simulink model "cameraCar_cs_mohammad"  (R2017b)
settings: Solver=ode5  StartTime=0.0  StopTime=inf  FixedStep=1/200  RelTol=1e-3
PreLoadFcn:
  | mbxruntime.callbacks.PreLoadFcn(bdroot);
PostLoadFcn:
  | mbxruntime.callbacks.PostLoadFcn(bdroot);
InitFcn:
  | mbxruntime.callbacks.InitFcn(bdroot);
StartFcn:
  | mbxruntime.callbacks.StartFcn(bdroot);
StopFcn:
  | mbxruntime.callbacks.StopFcn(bdroot);
model workspace (MAT data in the model file):
  mbox_table : struct (value not decoded)
  model_closed = 0
  sim_status = 0
undefined symbols (not defined in the file or in its folder): DiscIntNeverNeededParam, warningInitialVelocity, x0
libraries: simulink x19, dspnetwork x9, etargetslib x8, simulink_extras x5, PreScanSimulinkLibrary x4
(part 4 of 4)

== system cameraCar_cs_mohammad/Toyota_Yaris_Hatchback_1/Dynamics_Simple/Chassis/Bicycle_model_[XYZ]/Y & Yaw_Motion/Configurable Subsystem ==
  In1 : Inport
  In2 : Inport  Port=2
  Integrator : Integrator  ExternalReset=level
  Out1 : Outport
  wires:
  In1/1 -> Integrator/1
  In2/1 -> Integrator/2
  Integrator/1 -> Out1/1

== system cameraCar_cs_mohammad/Toyota_Yaris_Hatchback_1/Dynamics_Simple/Chassis/Bicycle_model_[XYZ]/Y & Yaw_Motion/Configurable Subsystem1 ==
  In1 : Inport
  Integrator : Integrator
  Out1 : Outport
  wires:
  In1/1 -> Integrator/1
  Integrator/1 -> Out1/1

== system cameraCar_cs_mohammad/Toyota_Yaris_Hatchback_1/Dynamics_Simple/Chassis/Bicycle_model_[XYZ]/Y & Yaw_Motion/Configurable Subsystem2 ==
  In1 : Inport
  In2 : Inport  Port=2
  Integrator : Integrator  ExternalReset=level
  Out1 : Outport
  wires:
  In1/1 -> Integrator/1
  In2/1 -> Integrator/2
  Integrator/1 -> Out1/1

== system cameraCar_cs_mohammad/Toyota_Yaris_Hatchback_1/Dynamics_Simple/Chassis/Bicycle_model_[XYZ]/Z, Pitch_Motion & Roll_Motion/Configurable Subsystem ==
  In1 : Inport
  Integrator : Integrator  LimitOutput=on  UpperSaturationLimit=5*pi/180  LowerSaturationLimit=-5*pi/180
  Out1 : Outport
  wires:
  In1/1 -> Integrator/1
  Integrator/1 -> Out1/1

== system cameraCar_cs_mohammad/Toyota_Yaris_Hatchback_1/Dynamics_Simple/Chassis/Bicycle_model_[XYZ]/Z, Pitch_Motion & Roll_Motion/Configurable Subsystem1 ==
  In1 : Inport
  Integrator : Integrator
  Out1 : Outport
  wires:
  In1/1 -> Integrator/1
  Integrator/1 -> Out1/1

== system cameraCar_cs_mohammad/Toyota_Yaris_Hatchback_1/Dynamics_Simple/Chassis/Bicycle_model_[XYZ]/Z, Pitch_Motion & Roll_Motion/Configurable Subsystem2 ==
  In1 : Inport
  Integrator : Integrator
  Out1 : Outport
  wires:
  In1/1 -> Integrator/1
  Integrator/1 -> Out1/1

== system cameraCar_cs_mohammad/Toyota_Yaris_Hatchback_1/Dynamics_Simple/Chassis/Bicycle_model_[XYZ]/Z, Pitch_Motion & Roll_Motion/Configurable Subsystem3 ==
  In1 : Inport
  Integrator : Integrator
  Out1 : Outport
  wires:
  In1/1 -> Integrator/1
  Integrator/1 -> Out1/1

== system cameraCar_cs_mohammad/Toyota_Yaris_Hatchback_1/Dynamics_Simple/Chassis/Bicycle_model_[XYZ]/Z, Pitch_Motion & Roll_Motion/Configurable Subsystem4 ==
  In1 : Inport
  Integrator : Integrator
  Out1 : Outport
  wires:
  In1/1 -> Integrator/1
  Integrator/1 -> Out1/1

== system cameraCar_cs_mohammad/Toyota_Yaris_Hatchback_1/Dynamics_Simple/Chassis/Bicycle_model_[XYZ]/Z, Pitch_Motion & Roll_Motion/Configurable Subsystem5 ==
  In1 : Inport
  Integrator : Integrator
  Out1 : Outport
  wires:
  In1/1 -> Integrator/1
  Integrator/1 -> Out1/1

== system cameraCar_cs_mohammad/Toyota_Yaris_Hatchback_1/Dynamics_Simple/Chassis/Bicycle_model_[XYZ]/Z, Pitch_Motion & Roll_Motion/Configurable Subsystem9 ==
  In1 : Inport
  Derivative : Derivative
  Out1 : Outport
  wires:
  In1/1 -> Derivative/1
  Derivative/1 -> Out1/1

== system cameraCar_cs_mohammad/Toyota_Yaris_Hatchback_1/Dynamics_Simple/Chassis/FrontTyre/AlphaFront/Enabled Subsystem ==
  In : Inport
  Enable : EnablePort  PropagateVarSize=During execution
  AlphaFront : Fcn  Expr=-atan( (u(2)+u(3)*p.a)/u(1) )
  Alpha : Outport  OutputWhenDisabled=reset  InitialOutput=[0]
  wires:
  AlphaFront/1 -> Alpha/1
  In/1 -> AlphaFront/1

== system cameraCar_cs_mohammad/Toyota_Yaris_Hatchback_1/Dynamics_Simple/Chassis/RearTyre/AlphaRear/Enabled Subsystem ==
  In : Inport
  Enable : EnablePort  PropagateVarSize=During execution
  AlphaRear : Fcn  Expr=-atan( (u(2)-u(3)*p.b)/u(1) )
  Alpha : Outport  OutputWhenDisabled=reset  InitialOutput=[0]
  wires:
  AlphaRear/1 -> Alpha/1
  In/1 -> AlphaRear/1

== system cameraCar_cs_mohammad/Toyota_Yaris_Hatchback_1/Dynamics_Simple/Chassis/Bicycle_model_[XYZ]/X_Motion/Max RPM and zero- velocity detection/Configurable Subsystem ==
  Step : Step  Time=0.0001  Before=1  After=0  SampleTime=0
  Out1 : Outport
  wires:
  Step/1 -> Out1/1

== system cameraCar_cs_mohammad/Toyota_Yaris_Hatchback_1/Dynamics_Simple/Chassis/Bicycle_model_[XYZ]/X_Motion/Max RPM and zero- velocity detection/SR-Memory ==
  Signal : Inport
  Set : Inport  Port=2
  Reset : Inport  Port=3
  Constant : Constant  Value=0
  Detect Rise Positive : simulink/Logic and Bit Operations/Detect Rise Positive  vinit=0  OutDataTypeStr=uint8
  Detect Rise Positive1 : simulink/Logic and Bit Operations/Detect Rise Positive  vinit=0  OutDataTypeStr=uint8
  Manual Switch : ManualSwitch
  Manual Switch1 : ManualSwitch
  Switch : Switch  Criteria=u2 ~= 0
  Switch1 : Switch  Criteria=u2 ~= 0
  Unit Delay : UnitDelay  SampleTime=-1
  Out : Outport
  wires:
  Constant/1 -> Switch1/1
  Switch/1 -> Switch1/3
  Switch1/1 -> Unit Delay/1, Out/1
  Manual Switch1/1 -> Switch1/2
  Reset/1 -> Manual Switch1/2, Detect Rise Positive1/1
  Detect Rise Positive1/1 -> Manual Switch1/1
  Signal/1 -> Switch/1
  Unit Delay/1 -> Switch/3
  Set/1 -> Detect Rise Positive/1, Manual Switch/2
  Detect Rise Positive/1 -> Manual Switch/1
  Manual Switch/1 -> Switch/2

== matlab function cameraCar_cs_mohammad/Toyota_Yaris_Hatchback_1/PathFollower_Preview_1/LateralController/CTRL REFERENCES/Calculate Lateral Error/eml_find_10k_lateral_error_points ==
  settings: updateMethod=DISCRETE
  data: pvp input size=2; dist_psvehicle output size=10; TrajOffset_x_y_Y input size=3; ActorOffset_Left_Right input; p0 input size=2; PreviewDistance input size=10; Traj_x parameter; Traj_y parameter; Traj_t parameter; Traj_v parameter; RefreshCounter parameter
function dist_psvehicle  = eml_find_10k_lateral_error_points(pvp,TrajOffset_x_y_Y,ActorOffset_Left_Right,p0,PreviewDistance,Traj_x,Traj_y,Traj_t,Traj_v,RefreshCounter)

dist_psvehicle = emlfcn_find_10k_lateral_error_points(pvp,TrajOffset_x_y_Y,ActorOffset_Left_Right,p0,PreviewDistance,Traj_x,Traj_y,Traj_t,Traj_v,RefreshCounter);

% end function

== matlab function cameraCar_cs_mohammad/Toyota_Yaris_Hatchback_1/Simulation time ==
  data: t input; y output
function y = fcn(t)

y =t; %s(4) is the 4th elements in the agent state: the host speed
%pause(1);

== matlab function cameraCar_cs_mohammad/Toyota_Yaris_Hatchback_1/PathFollower_Preview_1/LateralController/CTRL REFERENCES/Find Reference Point (pref0) on Trajectory closest to P0 Point (p0)/eml_find_closest_trajectory_points0 ==
  data: pvp input size=2; Actor_traj_distance output; TrajOffset_x_y_Y input size=3; ActorOffset_Left_Right input; p0 input size=3; Traj_x parameter; Traj_y parameter; Actor_traj_angle output; RefreshCounter parameter
function [Actor_traj_distance,Actor_traj_angle]  = eml_find_closest_trajectory_points0(pvp,TrajOffset_x_y_Y,ActorOffset_Left_Right,p0,Traj_x,Traj_y,RefreshCounter)

[Actor_traj_distance,Actor_traj_angle]  = emlfcn_find_closest_trajectory_points0(pvp,TrajOffset_x_y_Y,ActorOffset_Left_Right,p0,Traj_x,Traj_y,RefreshCounter);

% end function

== matlab function cameraCar_cs_mohammad/Toyota_Yaris_Hatchback_1/MATLAB Function2 ==
  data: u input; y output
function y = fcn(u)

y = u(1);

== matlab function cameraCar_cs_mohammad/Toyota_Yaris_Hatchback_1/PathFollower_Preview_1/LateralController/Calculate delta steering error/eml_delta_steering_error ==
  data: v_x_vehicle input; v_x_vehicle_Min input; t_Preview_LatCtrl input; delta_steeringwheeltotal output; v_y_vehicle input; yawrate_vehicle input; CorneringStiffness_Tyres_Front input; CorneringStiffness_Tyres_Rear input; m_vehicle_total input; inertia_z_vehicle_total input; e_Lat input size=10; Pos_x_CoG_Vehicle input; wheelbase input; RefreshCounter parameter
function delta_steeringwheeltotal = eml_delta_steering_error(v_x_vehicle,v_x_vehicle_Min,t_Preview_LatCtrl,v_y_vehicle,yawrate_vehicle,CorneringStiffness_Tyres_Front,CorneringStiffness_Tyres_Rear,m_vehicle_total,inertia_z_vehicle_total,e_Lat,Pos_x_CoG_Vehicle,wheelbase,RefreshCounter)

delta_steeringwheeltotal = emlfcn_delta_steering_error(v_x_vehicle,v_x_vehicle_Min,t_Preview_LatCtrl,v_y_vehicle,yawrate_vehicle,CorneringStiffness_Tyres_Front,CorneringStiffness_Tyres_Rear,m_vehicle_total,inertia_z_vehicle_total,e_Lat,Pos_x_CoG_Vehicle,wheelbase,RefreshCounter);

% end function

== matlab function cameraCar_cs_mohammad/Toyota_Yaris_Hatchback_1/Reward Calculator ==
  data: s input; R output
function R = fcn(s)

R =s(4); %s(4) is the 4th elements in the agent state: the host speed
%pause(1);

== matlab function cameraCar_cs_mohammad/Toyota_Yaris_Hatchback_1/position ==
  data: u input; y output
function y = fcn(u)
y = u(1);
%pause(1);

== matlab function cameraCar_cs_mohammad/Toyota_Yaris_Hatchback_1/json ==
  data: s input; y output
function y = fcn(s)
coder.extrinsic('num2str','bdroot','get_param');
p = 15;
s(isnan(s)) = 0;
u = (zeros(9,p));
m = (num2str(10*s(:), ['%0.' num2str(p) 'f ']));
sss = 1:p;
u(1,sss) = m(1,sss);    
u(2,sss) = m(2,sss);
u(3,sss) = m(3,sss);
u(4,sss) = m(4,sss);
u(5,sss) = m(5,sss);
u(6,sss) = m(6,sss);
u(7,sss) = m(7,sss);
u(8,sss) = m(8,sss);
u(9,sss) = m(9,sss);
t = num2str(round(get_param(bdroot,'SimulationTime'),p),['%0.' num2str(p) 'f ']);
ts = (32*ones(1,p));
ts(sss) = t(1,sss);

len = (89 + 9*p) + (8 + p);
y = uint8(32*ones(1,len));
y(1:end) = uint8(['{"Time":' ts ',"Position":{"x":' u(1,:) ',"y":' u(2,:) ',"z":' u(3,:) '},' ...
        '"Velocity":{"x":' u(4,:) ',"y":' u(5,:) ',"z":' u(6,:) '},' ...
        '"Acceleration":{"x":' u(7,:) ',"y":' u(8,:) ',"z":' u(9,:) '}}']);
y = uint8(y);
% json_s = string('{"Position":{"x":')+string(u(1))+string(',"y":')+string(u(2))+string(',"z":')+string(u(3))+string('},')+ string('"Velocity":{"x":')+string(u(4))+string(',"y":')+string(u(5))+string(',"z":')+string(u(6))+string('},')+ string('"Acceleration":{"x":')+string(u(7))+string(',"y":')+string(u(8))+string(',"z":')+string(u(9))+string('}}');
% json_s = string(5);
% y = char(json_s);
% y = struct('a',u(1));
% str = ['{"Position":{"x":' num2str(u(1)) ',"y":' num2str(u(2)) ',"z":' num2str(u(3)) '},' ...
%         '"Velocity":{"x":' num2str(u(4)) ',"y":' num2str(u(5)) ',"z":' num2str(u(6)) '},' ...
%         '"Acceleration":{"x":' num2str(u(7)) ',"y":' num2str(u(8)) ',"z":' num2str(u(9)) '}}'];
% u = udp('localhost',8090);
% fopen(u)
% %Send string over udp
% fwrite(u,str)
% fclose(u)

== matlab function cameraCar_cs_mohammad/Toyota_Yaris_Hatchback_1/speed ==
  data: u input; y output
function y = fcn(u)
y = u(4);
%pause(1);

== matlab function cameraCar_cs_mohammad/Toyota_Yaris_Hatchback_1/MATLAB Function3 ==
  data: u input; y output
function y = fcn(u)

y = u(1);

== matlab function cameraCar_cs_mohammad/Toyota_Yaris_Hatchback_1/MATLAB Function4 ==
  data: u input; y output
function y = fcn(u)

y = u(1);

== matlab function cameraCar_cs_mohammad/Toyota_Yaris_Hatchback_1/MATLAB Function5 ==
  data: u input; y output
function y = fcn(u)

y = u(1);

== matlab function cameraCar_cs_mohammad/Toyota_Yaris_Hatchback_1/MATLABFunction6 ==
  data: x input; y output
function y = fcn(x)

coder.extrinsic('set_param')
%coder.extrinsic('bdroot')
coder.extrinsic('sim')
  
y = 0;

if (x>671) 
    set_param('PreScan_Vissim_Python_0_cs', 'SimulationCommand', 'stop');
    y = 1;
end
